simulink model "scattering_vel"  (R2021a)
settings: Solver=FixedStepAuto  StartTime=0.0  StopTime=10  FixedStep=0.001  RelTol=1e-3
values from neighbouring files (symbols this model uses):
  B = 1    [scattering_params.m]    (also in scattering_params_vel.m)
  Be = 100    [scattering_params.m]    (also in scattering_params_vel.m = 15)
  Bh = 1.5    [scattering_params.m]    (also in scattering_params_vel.m = 70)
  Bm = 5    [scattering_params.m]    (also in scattering_params_vel.m = 1)
  Bs = 100    [scattering_params.m]    (also in scattering_params_vel.m = 5)
  Dh = 0.45    [scattering_params.m]    (also in scattering_params_vel.m = 10)
  Dm = 0    [scattering_params.m]    (also in scattering_params_vel.m)
  Ds = 0    [scattering_params.m]    (also in scattering_params_vel.m)
  Je = 0    [scattering_params.m]    (also in scattering_params_vel.m)
  Jh = 0.05    [scattering_params.m]    (also in scattering_params_vel.m)
  Ke = 200    [scattering_params.m]    (also in scattering_params_vel.m = 50)
  Kh = 1    [scattering_params.m]    (also in scattering_params_vel.m = 200)
  Km = 0.1    [scattering_params.m]    (also in scattering_params_vel.m = 5)
  Ks = 20    [scattering_params.m]    (also in scattering_params_vel.m = 140)
  Mm = 0.5    [scattering_params.m]    (also in scattering_params_vel.m)
  Ms = 2    [scattering_params.m]    (also in scattering_params_vel.m)
  Ph = 2    [scattering_params.m]    (also in scattering_params_vel.m = 55)
  Ts = 0.001    [scattering_params.m]    (also in scattering_params_vel.m)
undefined symbols (not defined in the file or in its folder): tau
libraries: simulink x5
settings Model: Creator=anuj  LastModifiedBy=antoninoparisi
settings DebuggingCC: SFMachineParentedDataDiag=warning

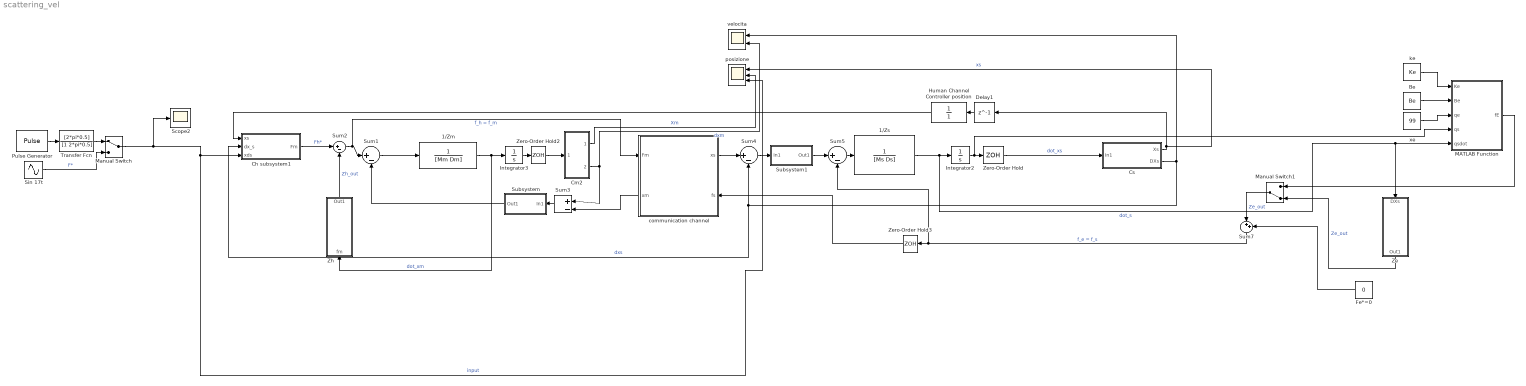
== system scattering_vel ==
  1/Zm : TransferFcn  Denominator=[Mm Dm]
  1/Zs : TransferFcn  Denominator=[Ms Ds]
  Be : Constant  Value=Be
  Ch subsystem1 : Subsystem
  Cm2 : Subsystem
  Cs : Subsystem
  Delay1 : Delay  DelayLength=1  SampleTime=Ts
  Fe*=0 : Constant  Value=0
  Human Channel Controller position : TransferFcn  Denominator=[1]
  Integrator2 : Integrator
  Integrator3 : Integrator
  MATLAB Function : MATLAB Function  TreatAsAtomicUnit=on
  Manual Switch : ManualSwitch
  Manual Switch1 : ManualSwitch  CurrentSetting=0
  Pulse Generator : DiscretePulseGenerator  PulseType=Time based  Period=10  PulseWidth=50  PhaseDelay=1
  Scope2 : Scope
  Sin 17t : Sin  Amplitude=0.5  Frequency=2*pi*1  SampleTime=0
  Subsystem : Subsystem
  Subsystem1 : Subsystem
  Sum{1..5} (5 alike) : Sum  Inputs=|+-
  Sum7 : Sum  Inputs=|++
  Transfer Fcn : TransferFcn  Numerator=[2*pi*0.5]  Denominator=[1 2*pi*0.5]
  Ze : Subsystem
  Zero-Order Hold : ZeroOrderHold  SampleTime=-1
  Zero-Order Hold2 : ZeroOrderHold  SampleTime=-1
  Zero-Order Hold3 : ZeroOrderHold  SampleTime=Ts
  Zh : Subsystem
  communication channel : Subsystem
      settings: PortSchema="{\"entries\":[{\"content\":{\"sides\":[{\"content\":{\"connectorIds\":[\"In1\",\"Out2\"]},\"type\":\"ConnectorPlacement.EquallySpacedRectSide\",\"uuid\":\"e201856c-da4b-4980-a88b-c6c86de05881\"},{\"content\":{\"connectorIds\":[\"Out1\",\"In2\"],\"side\":\"RIGHT\"},\"type\":\"ConnectorPlacement.EquallySpacedRectSide\",\"uuid\":\"94e31da8-7242-4dd7-9573-e1ea0d94f21a\"},{\"content\":{\"connectorIds\":[],\"side\":\"TOP\"},\"type\":\"ConnectorPlacement.EquallySpacedRectSide\",\"uuid\":\"bf228117-dafc-454a-bb50-819d6ba8707f\"}]},\"type\":\"ConnectorPlacement.EquallySpacedConnector\",\"uuid\":\"7a0eb8a2-b25a-4eac-8153-08b01a29f1b4\"}],\"packageUris\":[\"http://schema.mathworks.com/mf0/Connector/R2020b\"],\"version\":\"1.0\"}"
  ke : Constant  Value=Ke
  posizione : Scope  NumInputPorts=3
  velocita : Scope  NumInputPorts=2
  xe : Constant  Value=99
  wires:
  Sum2/1 -> communication channel/1(Fm), Sum1/1  "f_h = f_m"
  Manual Switch1/1 -> Sum7/1  "Ze_out"
  Ch subsystem1/1(Fm) -> Sum2/1  "Fh*"
  MATLAB Function/1(fE) -> Manual Switch1/1
  1/Zm/1 -> Zh/1(fm), Integrator3/1  "dot_xm"
  Sum1/1 -> 1/Zm/1
  Human Channel Controller position/1 -> Ch subsystem1/1(xs)
  Be/1 -> MATLAB Function/2(Be)
  Cs/1(Xs) -> Delay1/1, posizione/1  "xs"
  Fe*=0/1 -> Sum7/2
  xe/1 -> MATLAB Function/3(qe)
  ke/1 -> MATLAB Function/1(Ke)
  Manual Switch/1 -> posizione/3, Ch subsystem1/3(xds), Scope2/1  "input"
  Zh/1(Out1) -> Sum2/2  "Zh_out"
  Ze/1(Out1) -> Manual Switch1/2  "Ze_out"
  Zero-Order Hold/1 -> Cs/1(In1)  "dot_xs"
  Integrator2/1 -> MATLAB Function/4(qs), Zero-Order Hold/1
  Integrator3/1 -> Zero-Order Hold2/1
  Zero-Order Hold2/1 -> Cm2/1(In1)
  Sum7/1 -> Sum5/2, Zero-Order Hold3/1  "f_e = f_s"
  Zero-Order Hold3/1 -> communication channel/2(fs)
  Cs/2(DXs) -> velocita/1, Sum4/2, Ch subsystem1/2(dx_s)  "dxs"
  1/Zs/1 -> MATLAB Function/5(qsdot), Ze/1(DXs), Integrator2/1  "dot_s"
  Delay1/1 -> Human Channel Controller position/1
  Pulse Generator/1 -> Transfer Fcn/1
  Transfer Fcn/1 -> Manual Switch/1
  Sin 17t/1 -> Manual Switch/2  "F*"
  Cm2/2(DXm) -> velocita/2, Sum3/1  "dxm"
  communication channel/1(xs) -> Sum4/1
  Sum5/1 -> 1/Zs/1
  Cm2/1(Xm) -> posizione/2  "Xm"
  Subsystem/1(Out1) -> Sum1/2
  communication channel/2(xm) -> Sum3/2
  Sum3/1 -> Subsystem/1(In1)
  Sum4/1 -> Subsystem1/1(In1)
  Subsystem1/1(Out1) -> Sum5/1

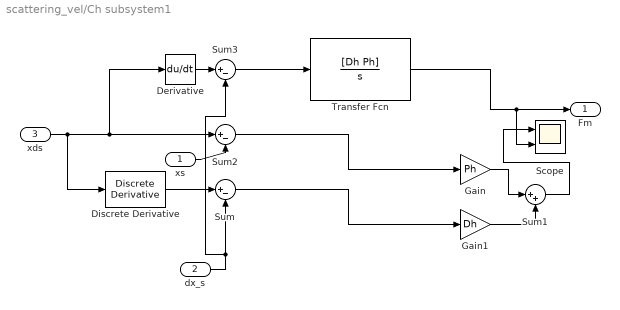
== system scattering_vel/Ch subsystem1 ==
  xs : Inport
  dx_s : Inport  Port=2
  xds : Inport  Port=3
  Derivative : Derivative
  Discrete Derivative : simulink/Discrete/Discrete Derivative  gainval=1.0  ICPrevScaledInput=0.0  OutMin=[]  OutMax=[]  OutDataType=fixdt(1, 16)  OutScaling=2^-10  DoSatur=off
  Gain : Gain  Gain=Ph
  Gain1 : Gain  Gain=Dh
  Scope : Scope  NumInputPorts=2
  Sum : Sum  Inputs=|+-
  Sum1 : Sum  Inputs=|++
  Sum2 : Sum  Inputs=|+-
  Sum3 : Sum  Inputs=|+-
  Transfer Fcn : TransferFcn  Numerator=[Dh Ph]  Denominator=[1 0]
  Fm : Outport
  wires:
  Gain1/1 -> Sum1/2
  Gain/1 -> Sum1/1
  xs/1 -> Sum2/2
  Discrete Derivative/1 -> Sum/1
  Sum/1 -> Gain1/1
  Sum2/1 -> Gain/1
  xds/1 -> Derivative/1, Sum2/1, Discrete Derivative/1
  dx_s/1 -> Sum3/2, Sum/2
  Derivative/1 -> Sum3/1
  Sum3/1 -> Transfer Fcn/1
  Transfer Fcn/1 -> Scope/2, Fm/1
  Sum1/1 -> Scope/1

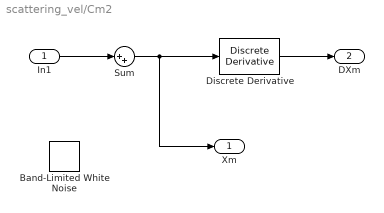
== system scattering_vel/Cm2 ==
  In1 : Inport
  Band-Limited White Noise : simulink/Sources/Band-Limited White Noise  Cov=[0.0000001]  Ts=Ts  seed=[23341]
  Discrete Derivative : simulink/Discrete/Discrete Derivative  gainval=1.0  ICPrevScaledInput=0.0  OutMin=[]  OutMax=[]  OutDataType=fixdt(1, 16)  OutScaling=2^-10  DoSatur=off
  Sum : Sum  Inputs=|++
  Xm : Outport
  DXm : Outport  Port=2
  wires:
  Sum/1 -> Xm/1, Discrete Derivative/1
  Discrete Derivative/1 -> DXm/1
  In1/1 -> Sum/1

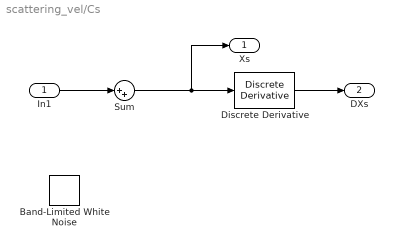
== system scattering_vel/Cs ==
  In1 : Inport
  Band-Limited White Noise : simulink/Sources/Band-Limited White Noise  Cov=[0.0000001]  Ts=Ts  seed=[23341]
  Discrete Derivative : simulink/Discrete/Discrete Derivative  gainval=1.0  ICPrevScaledInput=0.0  OutMin=[]  OutMax=[]  OutDataType=fixdt(1, 16)  OutScaling=2^-10  DoSatur=off
  Sum : Sum  Inputs=|++
  Xs : Outport
  DXs : Outport  Port=2
  wires:
  Sum/1 -> Xs/1, Discrete Derivative/1
  Discrete Derivative/1 -> DXs/1
  In1/1 -> Sum/1

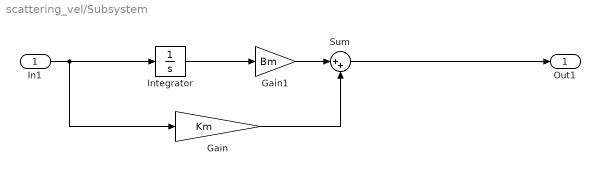
== system scattering_vel/Subsystem ==
  In1 : Inport
  Gain : Gain  Gain=Km
  Gain1 : Gain  Gain=Bm
  Integrator : Integrator
  Sum : Sum  Inputs=|++
  Out1 : Outport
  wires:
  In1/1 -> Integrator/1, Gain/1
  Gain1/1 -> Sum/1
  Gain/1 -> Sum/2
  Sum/1 -> Out1/1
  Integrator/1 -> Gain1/1

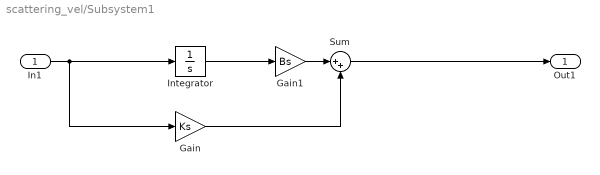
== system scattering_vel/Subsystem1 ==
  In1 : Inport
  Gain : Gain  Gain=Ks
  Gain1 : Gain  Gain=Bs
  Integrator : Integrator
  Sum : Sum  Inputs=|++
  Out1 : Outport
  wires:
  In1/1 -> Integrator/1, Gain/1
  Gain/1 -> Sum/2
  Sum/1 -> Out1/1
  Gain1/1 -> Sum/1
  Integrator/1 -> Gain1/1

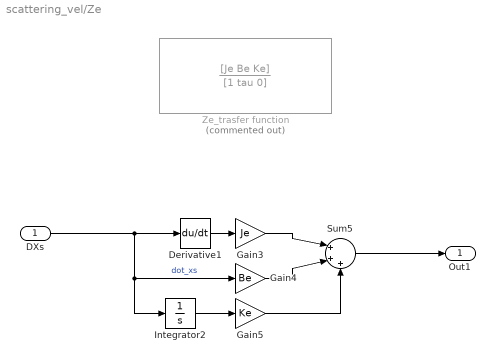
== system scattering_vel/Ze ==
  DXs : Inport
  Derivative1 : Derivative
  Gain3 : Gain  Gain=Je
  Gain4 : Gain  Gain=Be
  Gain5 : Gain  Gain=Ke
  Integrator2 : Integrator
  Sum5 : Sum  Inputs=|+++
  Ze_trasfer function : TransferFcn  Commented=on  Numerator=[Je Be Ke]  Denominator=[1 tau 0]
  Out1 : Outport
  wires:
  Gain4/1 -> Sum5/2
  Gain3/1 -> Sum5/1
  Gain5/1 -> Sum5/3
  Sum5/1 -> Out1/1
  Integrator2/1 -> Gain5/1
  DXs/1 -> Integrator2/1, Gain4/1, Derivative1/1  "dot_xs"
  Derivative1/1 -> Gain3/1

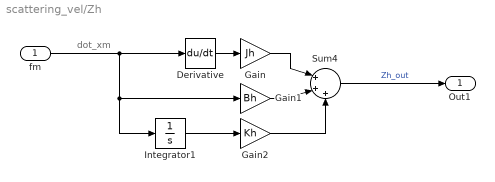
== system scattering_vel/Zh ==
  note: dot_xm
  fm : Inport
  Derivative : Derivative
  Gain : Gain  Gain=Jh
  Gain1 : Gain  Gain=Bh
  Gain2 : Gain  Gain=Kh
  Integrator1 : Integrator
  Sum4 : Sum  Inputs=|+++
  Out1 : Outport
  wires:
  Derivative/1 -> Gain/1
  Integrator1/1 -> Gain2/1
  Gain2/1 -> Sum4/3
  Gain1/1 -> Sum4/2
  Gain/1 -> Sum4/1
  Sum4/1 -> Out1/1  "Zh_out"
  fm/1 -> Gain1/1, Integrator1/1, Derivative/1

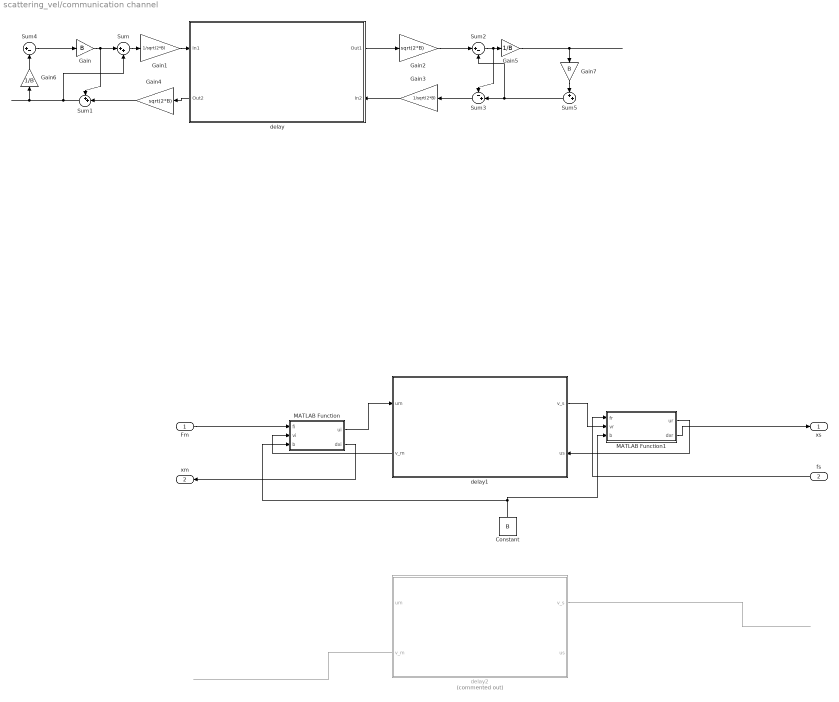
== system scattering_vel/communication channel ==
  Fm : Inport
  fs : Inport  Port=2
  Constant : Constant  Value=B
  Gain : Gain  Gain=B
  Gain1 : Gain  Gain=1/sqrt(2*B)
  Gain2 : Gain  Gain=sqrt(2*B)
  Gain3 : Gain  Gain=1/sqrt(2*B)
  Gain4 : Gain  Gain=sqrt(2*B)
  Gain5 : Gain  Gain=1/B
  Gain6 : Gain  Gain=1/B
  Gain7 : Gain  Gain=B
  MATLAB Function : MATLAB Function  TreatAsAtomicUnit=on
  MATLAB Function1 : MATLAB Function  TreatAsAtomicUnit=on
  Sum : Sum  Inputs=|++
  Sum1 : Sum  Inputs=++|
  Sum2 : Sum  Inputs=|+-
  Sum3 : Sum  Inputs=-+|
  Sum4 : Sum  Inputs=|+-
  Sum5 : Sum  Inputs=++|
  delay : Subsystem
      settings: PortSchema="{\"entries\":[{\"content\":{\"sides\":[{\"content\":{\"connectorIds\":[\"In1\",\"Out2\"]},\"type\":\"ConnectorPlacement.EquallySpacedRectSide\",\"uuid\":\"e201856c-da4b-4980-a88b-c6c86de05881\"},{\"content\":{\"connectorIds\":[\"Out1\",\"In2\"],\"side\":\"RIGHT\"},\"type\":\"ConnectorPlacement.EquallySpacedRectSide\",\"uuid\":\"94e31da8-7242-4dd7-9573-e1ea0d94f21a\"},{\"content\":{\"connectorIds\":[],\"side\":\"TOP\"},\"type\":\"ConnectorPlacement.EquallySpacedRectSide\",\"uuid\":\"bf228117-dafc-454a-bb50-819d6ba8707f\"}]},\"type\":\"ConnectorPlacement.EquallySpacedConnector\",\"uuid\":\"7a0eb8a2-b25a-4eac-8153-08b01a29f1b4\"}],\"packageUris\":[\"http://schema.mathworks.com/mf0/Connector/R2020b\"],\"version\":\"1.0\"}"
  delay1 : Subsystem
      settings: PortSchema="{\"entries\":[{\"content\":{\"sides\":[{\"content\":{\"connectorIds\":[\"In1\",\"Out2\"]},\"type\":\"ConnectorPlacement.EquallySpacedRectSide\",\"uuid\":\"e201856c-da4b-4980-a88b-c6c86de05881\"},{\"content\":{\"connectorIds\":[\"Out1\",\"In2\"],\"side\":\"RIGHT\"},\"type\":\"ConnectorPlacement.EquallySpacedRectSide\",\"uuid\":\"94e31da8-7242-4dd7-9573-e1ea0d94f21a\"},{\"content\":{\"connectorIds\":[],\"side\":\"TOP\"},\"type\":\"ConnectorPlacement.EquallySpacedRectSide\",\"uuid\":\"bf228117-dafc-454a-bb50-819d6ba8707f\"}]},\"type\":\"ConnectorPlacement.EquallySpacedConnector\",\"uuid\":\"7a0eb8a2-b25a-4eac-8153-08b01a29f1b4\"}],\"packageUris\":[\"http://schema.mathworks.com/mf0/Connector/R2020b\"],\"version\":\"1.0\"}"
  delay2 : Subsystem  Commented=on
      settings: PortSchema="{\"entries\":[{\"content\":{\"sides\":[{\"content\":{\"connectorIds\":[\"In1\",\"Out2\"]},\"type\":\"ConnectorPlacement.EquallySpacedRectSide\",\"uuid\":\"e201856c-da4b-4980-a88b-c6c86de05881\"},{\"content\":{\"connectorIds\":[\"Out1\",\"In2\"],\"side\":\"RIGHT\"},\"type\":\"ConnectorPlacement.EquallySpacedRectSide\",\"uuid\":\"94e31da8-7242-4dd7-9573-e1ea0d94f21a\"},{\"content\":{\"connectorIds\":[],\"side\":\"TOP\"},\"type\":\"ConnectorPlacement.EquallySpacedRectSide\",\"uuid\":\"bf228117-dafc-454a-bb50-819d6ba8707f\"}]},\"type\":\"ConnectorPlacement.EquallySpacedConnector\",\"uuid\":\"7a0eb8a2-b25a-4eac-8153-08b01a29f1b4\"}],\"packageUris\":[\"http://schema.mathworks.com/mf0/Connector/R2020b\"],\"version\":\"1.0\"}"
  xs : Outport
  xm : Outport  Port=2
  wires:
  Constant/1 -> MATLAB Function/3(b), MATLAB Function1/3(b)
  MATLAB Function/1(ui) -> delay1/1(um)
  MATLAB Function/2(dxi) -> xm/1
  delay1/1(v_s) -> MATLAB Function1/2(vr)
  MATLAB Function1/1(ur) -> delay1/2(us)
  MATLAB Function1/2(dxr) -> xs/1
  Sum1/1 -> Sum/2, Gain6/1
  Sum4/1 -> Gain/1
  ? -> Sum4/1
  Gain5/1 -> Gain7/1
  Sum5/1 -> Sum3/2, Sum2/2
  Gain/1 -> Sum1/1, Sum/1
  Sum/1 -> Gain1/1
  Gain1/1 -> delay/1(In1)
  delay/2(Out2) -> Gain4/1
  Sum3/1 -> Gain3/1
  Gain6/1 -> Sum4/2
  Gain2/1 -> Sum2/1
  Gain4/1 -> Sum1/2
  delay/1(Out1) -> Gain2/1
  ? -> Sum5/2
  Gain3/1 -> delay/2(In2)
  Gain7/1 -> Sum5/1
  Sum2/1 -> Sum3/1, Gain5/1
  fs/1 -> MATLAB Function1/1(fr)
  Fm/1 -> MATLAB Function/1(fi)
  delay1/2(v_m) -> MATLAB Function/2(vi)
  ? -> delay2/1(um)
  delay2/2(v_m) -> ?
  ? -> delay2/2(us)
  delay2/1(v_s) -> ?

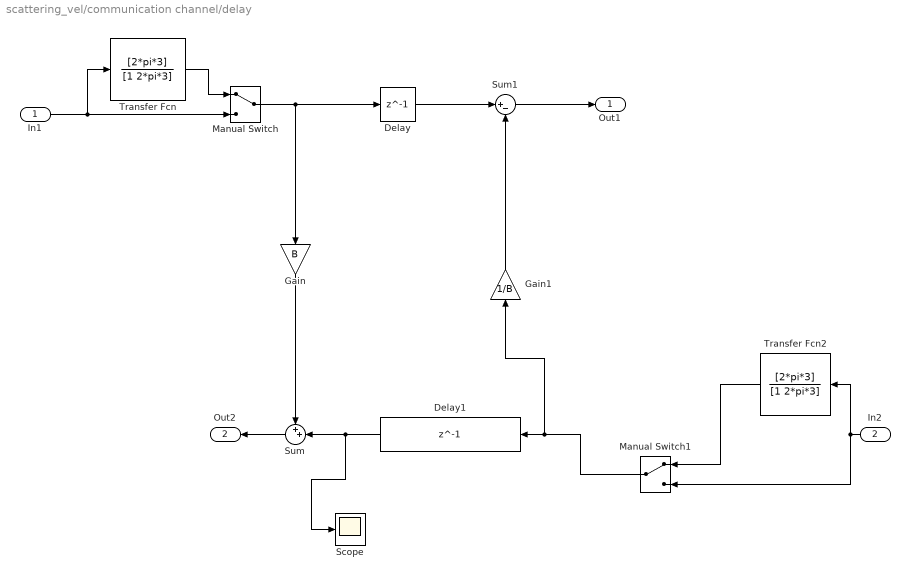
== system scattering_vel/communication channel/delay ==
  In1 : Inport
  In2 : Inport  Port=2
  Delay : Delay  DelayLength=1  InitialCondition=0
  Delay1 : Delay  DelayLength=1  InitialCondition=0
  Gain : Gain  Gain=B
  Gain1 : Gain  Gain=1/B
  Manual Switch : ManualSwitch
  Manual Switch1 : ManualSwitch
  Scope : Scope
  Sum : Sum  Inputs=++|
  Sum1 : Sum  Inputs=|+-
  Transfer Fcn : TransferFcn  Numerator=[2*pi*3]  Denominator=[1 2*pi*3]
  Transfer Fcn2 : TransferFcn  Numerator=[2*pi*3]  Denominator=[1 2*pi*3]
  Out1 : Outport
  Out2 : Outport  Port=2
  wires:
  Sum/1 -> Out2/1
  Gain/1 -> Sum/1
  Gain1/1 -> Sum1/2
  Sum1/1 -> Out1/1
  Delay/1 -> Sum1/1
  Delay1/1 -> Scope/1, Sum/2
  In1/1 -> Transfer Fcn/1, Manual Switch/2
  Transfer Fcn/1 -> Manual Switch/1
  Manual Switch/1 -> Gain/1, Delay/1
  Transfer Fcn2/1 -> Manual Switch1/1
  In2/1 -> Transfer Fcn2/1, Manual Switch1/2
  Manual Switch1/1 -> Gain1/1, Delay1/1

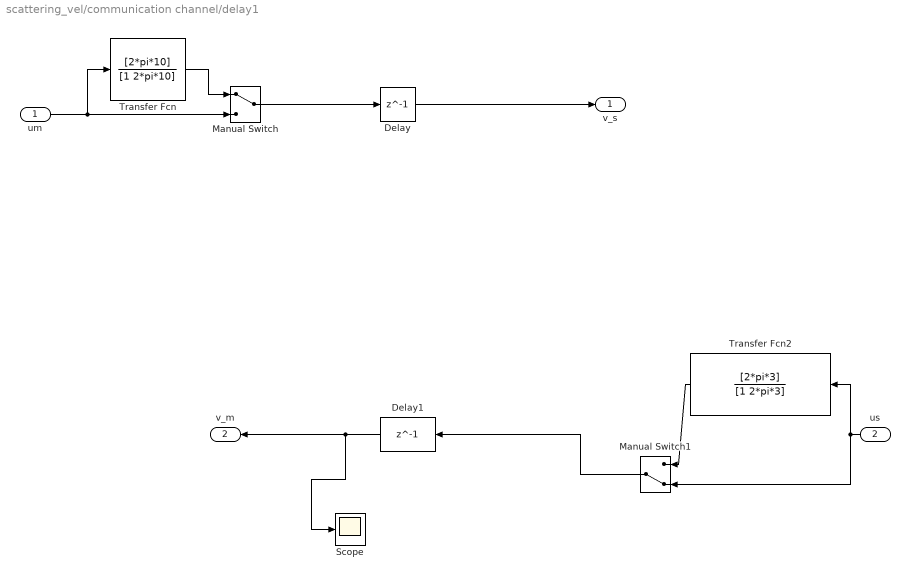
== system scattering_vel/communication channel/delay1 ==
  um : Inport
  us : Inport  Port=2
  Delay : Delay  DelayLength=1  InitialCondition=0  SampleTime=Ts
  Delay1 : Delay  DelayLength=1  InitialCondition=0  SampleTime=Ts
  Manual Switch : ManualSwitch
  Manual Switch1 : ManualSwitch  CurrentSetting=0
  Scope : Scope
  Transfer Fcn : TransferFcn  Numerator=[2*pi*10]  Denominator=[1 2*pi*10]
  Transfer Fcn2 : TransferFcn  Numerator=[2*pi*3]  Denominator=[1 2*pi*3]
  v_s : Outport
  v_m : Outport  Port=2
  wires:
  Delay1/1 -> v_m/1, Scope/1
  Delay/1 -> v_s/1
  um/1 -> Transfer Fcn/1, Manual Switch/2
  Transfer Fcn/1 -> Manual Switch/1
  Manual Switch/1 -> Delay/1
  Transfer Fcn2/1 -> Manual Switch1/1
  us/1 -> Transfer Fcn2/1, Manual Switch1/2
  Manual Switch1/1 -> Delay1/1

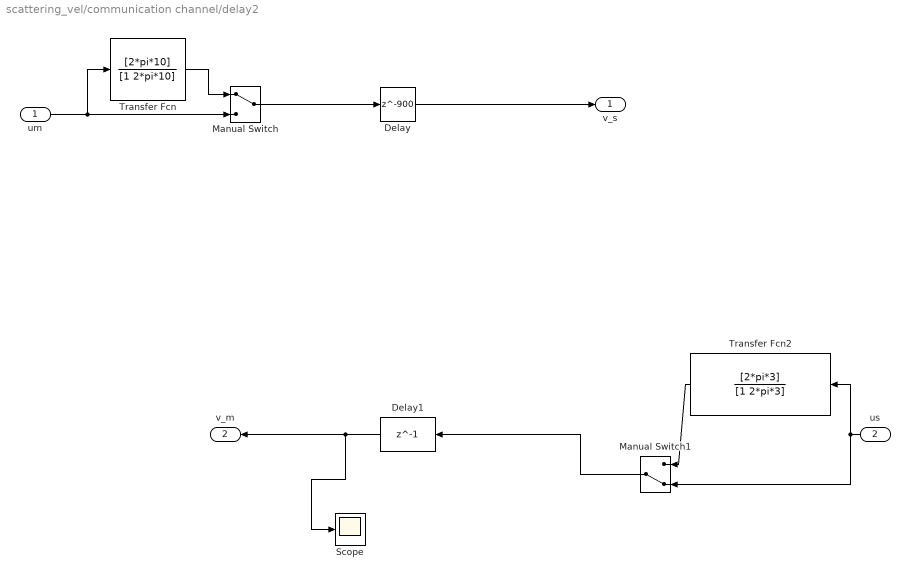
== system scattering_vel/communication channel/delay2 ==
  um : Inport
  us : Inport  Port=2
  Delay : Delay  DelayLength=900  InitialCondition=0  SampleTime=Ts
  Delay1 : Delay  DelayLength=1  InitialCondition=0  SampleTime=Ts
  Manual Switch : ManualSwitch
  Manual Switch1 : ManualSwitch  CurrentSetting=0
  Scope : Scope
  Transfer Fcn : TransferFcn  Numerator=[2*pi*10]  Denominator=[1 2*pi*10]
  Transfer Fcn2 : TransferFcn  Numerator=[2*pi*3]  Denominator=[1 2*pi*3]
  v_s : Outport
  v_m : Outport  Port=2
  wires:
  Delay1/1 -> v_m/1, Scope/1
  Delay/1 -> v_s/1
  um/1 -> Transfer Fcn/1, Manual Switch/2
  Transfer Fcn/1 -> Manual Switch/1
  Manual Switch/1 -> Delay/1
  Transfer Fcn2/1 -> Manual Switch1/1
  us/1 -> Transfer Fcn2/1, Manual Switch1/2
  Manual Switch1/1 -> Delay1/1

== matlab function scattering_vel/communication channel/MATLAB Function ==
  data: fi input; vi input; ui output; b input; dxi output
function [ui,dxi] = fcn(fi,vi,b)

ui = sqrt(2/b)*fi - vi;
dxi = 1/b*(fi - sqrt(2*b)*vi);
end

== matlab function scattering_vel/MATLAB Function ==
  data: Ke input; fE output; Be input; qe input; qs input; qsdot input
function fE = environment(Ke, Be, qe, qs, qsdot)
    if qs > qe
        fE = Ke * (qs - qe) + Be * qsdot;
    else
        fE = 0;
    end
end

== matlab function scattering_vel/communication channel/MATLAB Function1 ==
  data: fr input; vr input; ur output; b input; dxr output
function [ur,dxr] = fcn(fr,vr,b)


ur = sqrt(2/b) * fr - vr;
dxr = -1/b*(fr - sqrt(2*b)*vr);
